simulink model "DTF"  (R2022a)
settings: Solver=FixedStepDiscrete  StartTime=0.0  StopTime=0.04  FixedStep=0.04  RelTol=1e-3
PreLoadFcn:
  | listing = dir;
  | if (contains([listing .name], 'TCAF')) && (contains([listing .name], 'MAP'))
  |     addpath('./TCAF', './MAP');
  |     addpath( genpath('./MAP') );
  | elseif (contains([listing .name], 'DTF.slx'))
  |     addpath('../TCAF', '../MAP');
  |     addpath( genpath('../MAP') );
  | else
  | end
  | 
  | load('BusStructureDTF.mat');
  | load('BusStructureWTPG.mat');
  | load('TRN\BusStructureTRN.mat');
InitFcn:
  | listing = dir;
  | if (contains([listing .name], 'TCAF')) && (contains([listing .name], 'MAP'))
  |     addpath('./TCAF', './MAP');
  |     addpath( genpath('./MAP') );
  | elseif (contains([listing .name], 'DTF.slx'))
  |     addpath('../TCAF', '../MAP');
  |     addpath( genpath('../MAP') );
  | else
  | end
  | 
  | load('BusStructureDTF.mat');
  | load('BusStructureWTPG.mat');
  | load('TRN\BusStructureTRN.mat');
StartFcn:
  | listing = dir;
  | if (contains([listing .name], 'TCAF')) && (contains([listing .name], 'MAP'))
  |     addpath('./TCAF', './MAP');
  |     addpath( genpath('./MAP') );
  | elseif (contains([listing .name], 'DTF.slx'))
  |     addpath('../TCAF', '../MAP');
  |     addpath( genpath('../MAP') );
  | else
  | end
  | 
  | load('BusStructureDTF.mat');
  | load('BusStructureWTPG.mat');
  | load('TRN\BusStructureTRN.mat');
values from neighbouring files (symbols this model uses):
  isFeasible = logsout{idx_WTPGDatapump}.Values.isFeasible.Data(ii,:)    [WTPG_SIM_AFTERPLOT.m]
undefined symbols (not defined in the file or in its folder): gLimitWarning, lowTFWarning, m, msdUsedWrap, referenceTrajectory, rideQualityWrap, s, selectedWrap, statusCode, valid, verticalGCommand
libraries: hdlsllib x15, simulink x2, aerolibconvert2 x2, simulink_extras x1
settings Model: Creator=ASCL  LastModifiedBy=ASCL
settings DataIOCC: SaveOutput=off  SignalLogging=off  DSMLogging=off  SaveTime=off  ReturnWorkspaceOutputs=off
settings OptimizationCC: BlockReduction=off  DefaultParameterBehavior=Inlined  UseDivisionForNetSlopeComputation=on  GainParamInheritBuiltInType=on  UseFloatMulNetSlope=on  ExpressionFolding=off  PassReuseOutputArgsAs=Individual arguments  ZeroExternalMemoryAtStartup=off  ZeroInternalMemoryAtStartup=off  EfficientFloat2IntCast=on  LifeSpan=inf  OptimizeBlockOrder=speed  DifferentSizesBufferReuse=on  EfficientTunableParamExpr=on
settings DebuggingCC: SignalInfNanChecking=warning  ReadBeforeWriteMsg=EnableAllAsWarning  WriteAfterWriteMsg=EnableAllAsError  WriteAfterReadMsg=EnableAllAsError  IntegerOverflowMsg=error  ParameterTunabilityLossMsg=error  UniqueDataStoreMsg=error  AssertControl=DisableAll  NonBusSignalsTreatedAsBus=error  SFInvalidInputDataAccessInChartInitDiag=error  SFTransitionOutsideNaturalParentDiag=error  SFUnreachableExecutionPathDiag=error  SFUndirectedBroadcastEventsDiag=error  IntegerSaturationMsg=error
settings HardwareCC: ProdBitPerPointer=32  ProdBitPerSizeT=32  ProdBitPerPtrDiffT=32  ProdLargestAtomicInteger=Long  ProdLargestAtomicFloat=Double  ProdEndianess=BigEndian  ProdWordSize=32  ProdLongLongMode=on  ProdHWDeviceType=Freescale->MPC83xx
settings ModelReferenceCC: ModelReferenceNumInstancesAllowed=Single
settings SFSimCC: CompileTimeRecursionLimit=0  EnableRuntimeRecursion=off  MATLABDynamicMemAlloc=off
settings RTWCC: SystemTargetFile=ert.tlc  TemplateMakefile=ert_default_tmf  GenerateReport=on  RTWUseSimCustomCode=on  BuildConfiguration=Faster Runs  IncludeHyperlinkInReport=on  LaunchReport=on  GenerateTraceInfo=on  GenerateTraceReport=on  GenerateTraceReportSl=on  GenerateTraceReportSf=on  GenerateTraceReportEml=on  GenerateCodeMetricsReport=on
settings CodeAppCC: ForceParamTrailComments=on  IgnoreCustomStorageClasses=off  OperatorAnnotations=on  SimulinkDataObjDesc=on  SFDataObjDesc=on  MATLABFcnDesc=on  InsertBlockDesc=on  StateflowObjectComments=on  MATLABSourceComments=on  EnableCustomComments=on  InlinedPrmAccess=Macros  ReqsInCode=on
settings ERTTargetCC: TargetLangStandard=C99 (ISO)  UtilityFuncGeneration=Shared location  GenerateSampleERTMain=on  IncludeMdlTerminateFcn=off  CombineSignalStateStructs=on  SuppressErrorStatus=on  SupportAbsoluteTime=off  SupportNonFinite=off  SupportComplex=off  SupportVariableSizeSignals=on  ParenthesesLevel=Standards  CastingMode=Standards  GenerateSharedConstants=off  InlinedParameterPlacement=NonHierarchical  ERTCustomFileTemplate=example_file_process.tlc  RateTransitionBlockCode=Function  PreserveIfCondition=on  ConvertIfToSwitch=off  EnableSignedLeftShifts=off  EnableSignedRightShifts=off

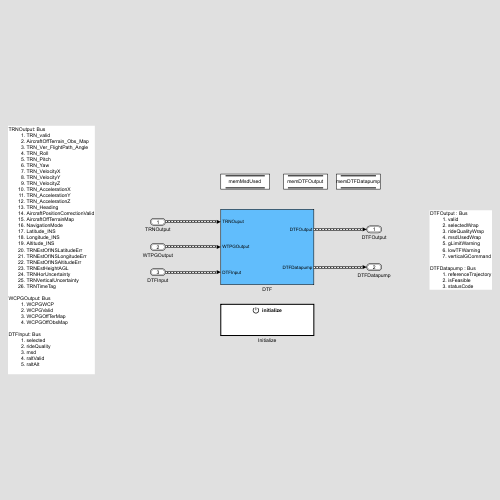
[thumbnail: Simulink's stored preview of the top-level diagram]
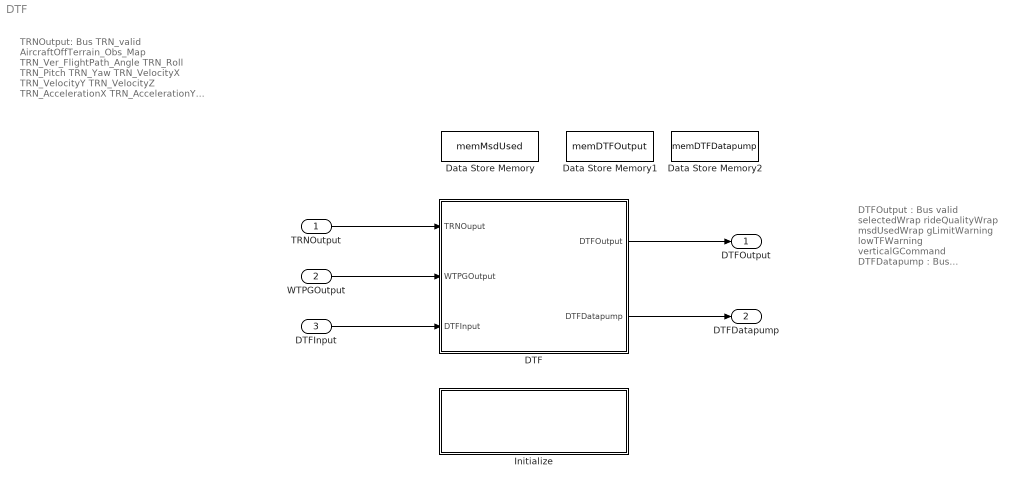
== system DTF ==
  note: TRNOutput: Bus
      | TRN_valid
      | AircraftOffTerrain_Obs_Map
      | TRN_Ver_FlightPath_Angle
      | TRN_Roll
      | TRN_Pitch
      | TRN_Yaw
      | TRN_VelocityX
      | TRN_VelocityY
      | TRN_VelocityZ
      | TRN_AccelerationX
      | TRN_AccelerationY
      | TRN_AccelerationZ
      | TRN_Heading
      | AircraftPositionCorrectionValid
      | AircraftOffTerrainMap
      | NavigationMode
      | Latitude_INS
      | Longitude_INS
      | Altitude_INS
      | TRNEstOfINSLatitudeErr
      | TRNEstOfINSLongitudeErr
      | TRNEstOfINSAltitudeErr
      | TRNEstHeightAGL
      | TRNHorUncertainty
      | TRNVerticalUncertainty
      | TRNTimeTag
      |
      | WCPGOutput: Bus
      | WCPGWCP
      | WCPGValid
      | WCPGOffTerMap
      | WCPGOffObsMap
      |
      | DTFInput: Bus
      | selected
      | rideQuality
      | msd
      | raltValid
      | raltAlt
  note: DTFOutput : Bus
      | valid
      | selectedWrap
      | rideQualityWrap
      | msdUsedWrap
      | gLimitWarning
      | lowTFWarning
      | verticalGCommand
      |
      | DTFDatapump : Bus
      | referenceTrajectory
      | isFeasible
      | statusCode
  TRNOutput : Inport  OutDataTypeStr=Bus: TRNOutput  Interpolate=off  BusOutputAsStruct=on
  WTPGOutput : Inport  Port=2  OutDataTypeStr=Bus: WTPGOutput  Interpolate=off  BusOutputAsStruct=on
  DTFInput : Inport  Port=3  OutDataTypeStr=Bus: DTFInput  Interpolate=off  BusOutputAsStruct=on
  DTF : Subsystem
  Data Store Memory : DataStoreMemory  DataStoreName=memMsdUsed  WriteAfterWriteMsg=warning  ShowAdditionalParam=off  OutDataTypeStr=double
      settings: LockScale=on
  Data Store Memory1 : DataStoreMemory  DataStoreName=memDTFOutput  WriteAfterWriteMsg=warning  ShowAdditionalParam=off  OutDataTypeStr=Bus: DTFOutput
      settings: LockScale=on
  Data Store Memory2 : DataStoreMemory  DataStoreName=memDTFDatapump  WriteAfterWriteMsg=warning  ShowAdditionalParam=off  OutDataTypeStr=Bus: DTFDatapump
      settings: LockScale=on
  Initialize : Subsystem  TreatAsAtomicUnit=on
  DTFOutput : Outport  OutDataTypeStr=Bus: DTFOutput  SampleTime=0.04  BusOutputAsStruct=on
  DTFDatapump : Outport  Port=2  OutDataTypeStr=Bus: DTFDatapump  SampleTime=0.04  BusOutputAsStruct=on
  wires:
  TRNOutput/1 -> DTF/1(TRNOuput)
  WTPGOutput/1 -> DTF/2(WTPGOutput)
  DTFInput/1 -> DTF/3(DTFInput)
  DTF/1(DTFOutput) -> DTFOutput/1
  DTF/2(DTFDatapump) -> DTFDatapump/1

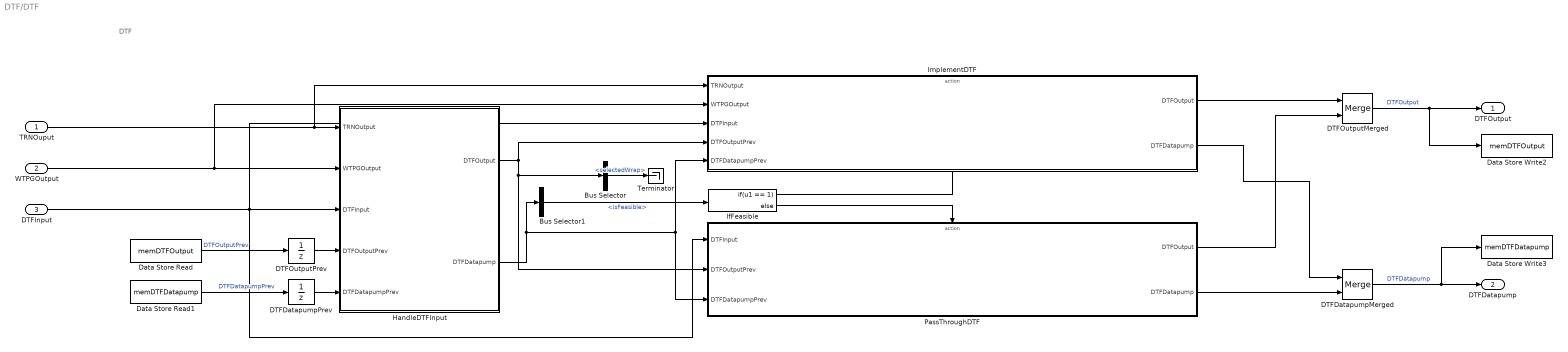
== system DTF/DTF ==
  note: DTF
  TRNOuput : Inport  OutDataTypeStr=Bus: TRNOutput
  WTPGOutput : Inport  Port=2  OutDataTypeStr=Bus: WTPGOutput
  DTFInput : Inport  Port=3  OutDataTypeStr=Bus: DTFInput
  Bus Selector : BusSelector  OutputSignals=selectedWrap
  Bus Selector1 : BusSelector  OutputSignals=isFeasible
  DTFDatapumpMerged : Merge
  DTFDatapumpPrev : UnitDelay  SampleTime=-1  HasFrameUpgradeWarning=on
  DTFOutputMerged : Merge
  DTFOutputPrev : UnitDelay  SampleTime=-1  HasFrameUpgradeWarning=on
  Data Store Read : DataStoreRead  DataStoreName=memDTFOutput  IndexOptions=Index vector (dialog)  Indices=1  OutputSizes=1
  Data Store Read1 : DataStoreRead  DataStoreName=memDTFDatapump  IndexOptions=Index vector (dialog)  Indices=1  OutputSizes=1
  Data Store Write2 : DataStoreWrite  DataStoreName=memDTFOutput  IndexOptions=Index vector (dialog)  Indices=1  OutputSizes=1
  Data Store Write3 : DataStoreWrite  DataStoreName=memDTFDatapump  IndexOptions=Index vector (dialog)  Indices=1  OutputSizes=1
  HandleDTFInput : Subsystem  TreatAsAtomicUnit=on
      settings: RTWSystemCode=Nonreusable function  RTWFcnNameOpts=Use subsystem name
  IfFeasible : If  IfExpression=u1 == 1
  ImplementDTF : Subsystem  TreatAsAtomicUnit=on
      settings: RTWSystemCode=Nonreusable function  RTWFcnNameOpts=Use subsystem name
  PassThroughDTF : Subsystem  TreatAsAtomicUnit=on
      settings: RTWSystemCode=Nonreusable function  RTWFcnNameOpts=Use subsystem name
  Terminator : Terminator
  DTFOutput : Outport  OutDataTypeStr=Bus: DTFOutput
  DTFDatapump : Outport  Port=2  OutDataTypeStr=Bus: DTFDatapump
  wires:
  ImplementDTF/1(DTFOutput) -> DTFOutputMerged/1
  PassThroughDTF/1(DTFOutput) -> DTFOutputMerged/2
  DTFOutputPrev/1 -> HandleDTFInput/4(DTFOutputPrev)
  IfFeasible/2 -> PassThroughDTF/Action
  TRNOuput/1 -> ImplementDTF/1(TRNOutput), HandleDTFInput/1(TRNOutput)
  Data Store Read/1 -> DTFOutputPrev/1  "DTFOutputPrev"
  DTFDatapumpPrev/1 -> HandleDTFInput/5(DTFDatapumpPrev)
  WTPGOutput/1 -> ImplementDTF/2(WTPGOutput), HandleDTFInput/2(WTPGOutput)
  ImplementDTF/2(DTFDatapump) -> DTFDatapumpMerged/1
  DTFInput/1 -> PassThroughDTF/1(DTFInput), ImplementDTF/3(DTFInput), HandleDTFInput/3(DTFInput)
  HandleDTFInput/2(DTFDatapump) -> Bus Selector1/1, PassThroughDTF/3(DTFDatapumpPrev), ImplementDTF/5(DTFDatapumpPrev)
  PassThroughDTF/2(DTFDatapump) -> DTFDatapumpMerged/2
  IfFeasible/1 -> ImplementDTF/Action
  Data Store Read1/1 -> DTFDatapumpPrev/1  "DTFDatapumpPrev"
  Bus Selector1/1 -> IfFeasible/1  "<isFeasible>"
  DTFOutputMerged/1 -> Data Store Write2/1, DTFOutput/1  "DTFOutput"
  DTFDatapumpMerged/1 -> Data Store Write3/1, DTFDatapump/1  "DTFDatapump"
  HandleDTFInput/1(DTFOutput) -> PassThroughDTF/2(DTFOutputPrev), Bus Selector/1, ImplementDTF/4(DTFOutputPrev)
  Bus Selector/1 -> Terminator/1  "<selectedWrap>"

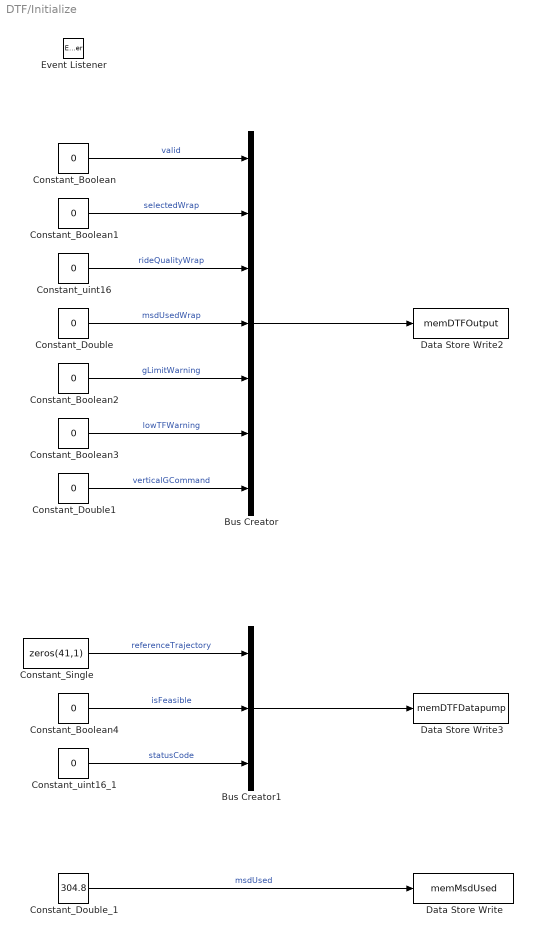
== system DTF/Initialize ==
  Bus Creator : BusCreator  Inputs=7  OutDataTypeStr=Bus: DTFOutput  NonVirtualBus=on
  Bus Creator1 : BusCreator  Inputs=3  OutDataTypeStr=Bus: DTFDatapump  NonVirtualBus=on
  Constant_Boolean{,1..4} (5 alike) : Constant  Value=0  OutDataTypeStr=boolean
  Constant_Double : Constant  Value=0  OutDataTypeStr=double
  Constant_Double1 : Constant  Value=0  OutDataTypeStr=double
  Constant_Double_1 : Constant  Value=304.8  VectorParams1D=off  OutDataTypeStr=double
  Constant_Single : Constant  Value=zeros(41,1)  OutDataTypeStr=single
  Constant_uint16 : Constant  Value=0  OutDataTypeStr=uint16
  Constant_uint16_1 : Constant  Value=0  OutDataTypeStr=uint16
  Data Store Write : DataStoreWrite  DataStoreName=memMsdUsed  IndexOptions=Index vector (dialog)  Indices=1  OutputSizes=1
  Data Store Write2 : DataStoreWrite  DataStoreName=memDTFOutput  IndexOptions=Index vector (dialog)  Indices=1  OutputSizes=1
  Data Store Write3 : DataStoreWrite  DataStoreName=memDTFDatapump  IndexOptions=Index vector (dialog)  Indices=1  OutputSizes=1
  Event Listener : EventListener  DisableCoverage=on  EventName=reset
  wires:
  Constant_Boolean/1 -> Bus Creator/1  "valid"
  Constant_Boolean1/1 -> Bus Creator/2  "selectedWrap"
  Constant_Boolean3/1 -> Bus Creator/6  "lowTFWarning"
  Constant_Boolean2/1 -> Bus Creator/5  "gLimitWarning"
  Constant_Double/1 -> Bus Creator/4  "msdUsedWrap"
  Constant_Double1/1 -> Bus Creator/7  "verticalGCommand"
  Constant_uint16/1 -> Bus Creator/3  "rideQualityWrap"
  Bus Creator/1 -> Data Store Write2/1
  Bus Creator1/1 -> Data Store Write3/1
  Constant_uint16_1/1 -> Bus Creator1/3  "statusCode"
  Constant_Boolean4/1 -> Bus Creator1/2  "isFeasible"
  Constant_Single/1 -> Bus Creator1/1  "referenceTrajectory"
  Constant_Double_1/1 -> Data Store Write/1  "msdUsed"

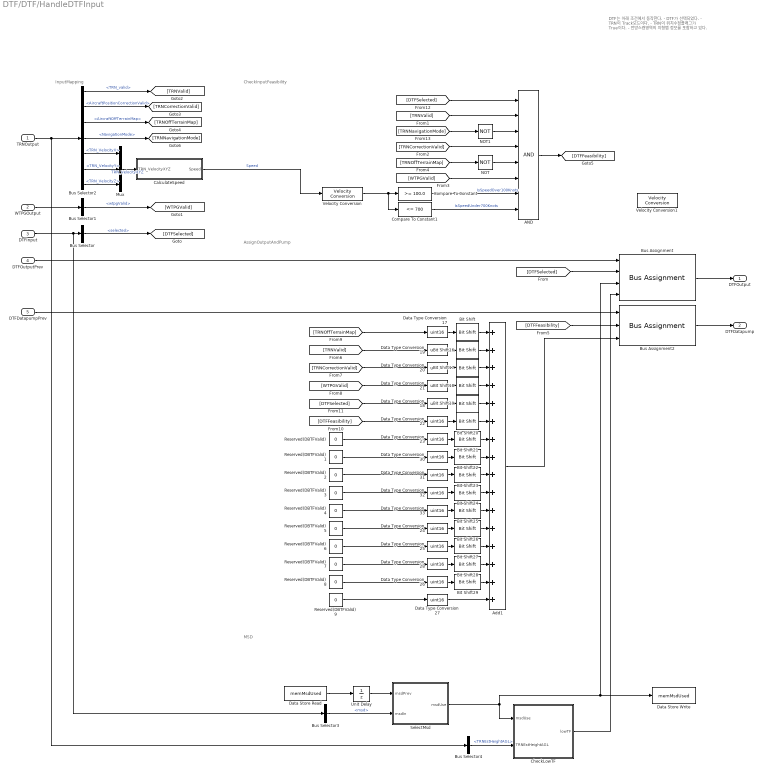
== system DTF/DTF/HandleDTFInput ==
  note: MSD
  note: AssignOutputAndPump
  note: DTF는 아래 조건에서 동작한다.
      | - DTF가 선택되었다.
      | - TRN이 Track모드이다.
      | - TRN이 위치수정플래그가 True이다.
      | - 전방스캔영역의 지형맵 정보를 포함하고 있다.
  note: CheckInputFeasibility
  note: InputMapping
  TRNOutput : Inport  OutDataTypeStr=Bus: TRNOutput
  WTPGOutput : Inport  Port=2  OutDataTypeStr=Bus: WTPGOutput
  DTFInput : Inport  Port=3  OutDataTypeStr=Bus: DTFInput
  DTFOutputPrev : Inport  Port=4  OutDataTypeStr=Bus: DTFOutput
  DTFDatapumpPrev : Inport  Port=5  OutDataTypeStr=Bus: DTFDatapump
  AND : Logic  Inputs=8  AllPortsSameDT=off  OutDataTypeStr=boolean
  Add1 : Sum  Inputs=++++++++++++++++  AccumDataTypeStr=uint16
  Bit Shift : hdlsllib/Logic and Bit Operations/Bit Shift  mode=Shift Left Logical  N=15
  Bit Shift16 : hdlsllib/Logic and Bit Operations/Bit Shift  mode=Shift Left Logical  N=14
  Bit Shift17 : hdlsllib/Logic and Bit Operations/Bit Shift  mode=Shift Left Logical  N=13
  Bit Shift18 : hdlsllib/Logic and Bit Operations/Bit Shift  mode=Shift Left Logical  N=12
  Bit Shift19 : hdlsllib/Logic and Bit Operations/Bit Shift  mode=Shift Left Logical  N=11
  Bit Shift20 : hdlsllib/Logic and Bit Operations/Bit Shift  mode=Shift Left Logical  N=10
  Bit Shift21 : hdlsllib/Logic and Bit Operations/Bit Shift  mode=Shift Left Logical  N=9
  Bit Shift22 : hdlsllib/Logic and Bit Operations/Bit Shift  mode=Shift Left Logical  N=8
  Bit Shift23 : hdlsllib/Logic and Bit Operations/Bit Shift  mode=Shift Left Logical  N=7
  Bit Shift24 : hdlsllib/Logic and Bit Operations/Bit Shift  mode=Shift Left Logical  N=6
  Bit Shift25 : hdlsllib/Logic and Bit Operations/Bit Shift  mode=Shift Left Logical  N=5
  Bit Shift26 : hdlsllib/Logic and Bit Operations/Bit Shift  mode=Shift Left Logical  N=4
  Bit Shift27 : hdlsllib/Logic and Bit Operations/Bit Shift  mode=Shift Left Logical  N=3
  Bit Shift28 : hdlsllib/Logic and Bit Operations/Bit Shift  mode=Shift Left Logical  N=2
  Bit Shift29 : hdlsllib/Logic and Bit Operations/Bit Shift  mode=Shift Left Logical  N=1
  Bus Assignment : BusAssignment  AssignedSignals=selectedWrap,msdUsedWrap,lowTFWarning
  Bus Assignment2 : BusAssignment  AssignedSignals=isFeasible,statusCode
  Bus Selector : BusSelector  OutputSignals=selected
  Bus Selector1 : BusSelector  OutputSignals=wtpgValid
  Bus Selector2 : BusSelector  OutputSignals=TRN_valid,AircraftPositionCorrectionValid,AircraftOffTerrainMap,NavigationMode,TRN_VelocityX,TRN_VelocityY,TRN_VelocityZ
  Bus Selector3 : BusSelector  OutputSignals=msd
  Bus Selector4 : BusSelector  OutputSignals=TRNEstHeightAGL
  CalculateSpeed : Subsystem
  CheckLowTF : MATLAB Function  TreatAsAtomicUnit=on
      settings: RTWSystemCode=Nonreusable function  RTWFcnNameOpts=Use subsystem name  FunctionInterfaceSpec=Allow arguments (Match graphical interface)
  Compare To Constant : simulink/Logic and Bit Operations/Compare To Constant  relop=>=  const=100.0  OutDataTypeStr=boolean
  Compare To Constant1 : simulink/Logic and Bit Operations/Compare To Constant  relop=<=  const=700  OutDataTypeStr=boolean
  Data Store Read : DataStoreRead  DataStoreName=memMsdUsed  IndexOptions=Index vector (dialog)  Indices=1  OutputSizes=1
  Data Store Write : DataStoreWrite  DataStoreName=memMsdUsed  IndexOptions=Index vector (dialog)  Indices=1  OutputSizes=1
  Data Type Conversion{17..28,30..33} (16 alike) : DataTypeConversion  OutDataTypeStr=uint16  SaturateOnIntegerOverflow=off  RndMeth=Floor
  Mux : Mux  Inputs=3
  NOT : Logic  Operator=NOT  AllPortsSameDT=off  OutDataTypeStr=boolean
  NOT1 : Logic  Operator=NOT  AllPortsSameDT=off  OutDataTypeStr=boolean
  Reserved(DBTFValid){,1..9} (10 alike) : Constant  Value=0  OutDataTypeStr=boolean
  SelectMsd : MATLAB Function  TreatAsAtomicUnit=on
      settings: RTWSystemCode=Nonreusable function  RTWFcnNameOpts=Use subsystem name  FunctionInterfaceSpec=Allow arguments (Match graphical interface)
  Unit Delay : UnitDelay  SampleTime=-1  HasFrameUpgradeWarning=on
  Velocity Conversion : aerolibconvert2/Velocity Conversion  IU=m/s  OU=kts
  Velocity Conversion1 : aerolibconvert2/Velocity Conversion  IU=m/s  OU=kts
  DTFOutput : Outport  OutDataTypeStr=Bus: DTFOutput  VectorParamsAs1DForOutWhenUnconnected=off
  DTFDatapump : Outport  Port=2  OutDataTypeStr=Bus: DTFDatapump  VectorParamsAs1DForOutWhenUnconnected=off
  wires:
  DTFInput/1 -> Bus Selector3/1, Bus Selector/1
  DTFOutputPrev/1 -> Bus Assignment/1
  Bus Assignment/1 -> DTFOutput/1
  DTFDatapumpPrev/1 -> Bus Assignment2/1
  WTPGOutput/1 -> Bus Selector1/1
  TRNOutput/1 -> Bus Selector4/1, Bus Selector2/1
  Bus Selector2/2 -> [TRNCorrectionValid]  "<AircraftPositionCorrectionValid>"
  Bus Selector2/3 -> [TRNOffTerrainMap]  "<AircraftOffTerrainMap>"
  Bus Selector/1 -> [DTFSelected]  "<selected>"
  Bus Selector1/1 -> [WTPGValid]  "<wtpgValid>"
  Bus Selector2/1 -> [TRNValid]  "<TRN_valid>"
  [DTFSelected] -> Bus Assignment/2
  [TRNOffTerrainMap] -> NOT/1
  Bus Assignment2/1 -> DTFDatapump/1
  Add1/1 -> Bus Assignment2/3
  [TRNOffTerrainMap] -> Data Type Conversion17/1
  [TRNCorrectionValid] -> Data Type Conversion20/1
  [WTPGValid] -> Data Type Conversion21/1
  [DTFFeasibility] -> Data Type Conversion22/1
  [DTFSelected] -> Data Type Conversion18/1
  Reserved(DBTFValid)/1 -> Data Type Conversion23/1
  [TRNValid] -> Data Type Conversion19/1
  AND/1 -> [DTFFeasibility]
  [DTFSelected] -> AND/1
  Bus Selector2/4 -> [TRNNavigationMode]  "<NavigationMode>"
  [TRNValid] -> AND/2
  [TRNNavigationMode] -> NOT1/1
  [TRNCorrectionValid] -> AND/4
  [WTPGValid] -> AND/6
  NOT/1 -> AND/5
  Data Type Conversion18/1 -> Bit Shift19/1
  Bit Shift/1 -> Add1/1
  Data Type Conversion27/1 -> Add1/16
  Data Type Conversion26/1 -> Bit Shift29/1
  Bit Shift29/1 -> Add1/15
  Data Type Conversion33/1 -> Bit Shift25/1
  Data Type Conversion22/1 -> Bit Shift20/1
  Data Type Conversion20/1 -> Bit Shift17/1
  Data Type Conversion24/1 -> Bit Shift26/1
  Data Type Conversion19/1 -> Bit Shift16/1
  Bit Shift28/1 -> Add1/14
  Data Type Conversion32/1 -> Bit Shift24/1
  Data Type Conversion23/1 -> Bit Shift21/1
  Bit Shift23/1 -> Add1/9
  Data Type Conversion25/1 -> Bit Shift27/1
  Data Type Conversion30/1 -> Bit Shift22/1
  Data Type Conversion17/1 -> Bit Shift/1
  Data Type Conversion31/1 -> Bit Shift23/1
  Bit Shift24/1 -> Add1/10
  Data Type Conversion28/1 -> Bit Shift28/1
  Bit Shift25/1 -> Add1/11
  Data Type Conversion21/1 -> Bit Shift18/1
  Bit Shift27/1 -> Add1/13
  Bit Shift21/1 -> Add1/7
  Bit Shift19/1 -> Add1/5
  Bit Shift20/1 -> Add1/6
  Bit Shift22/1 -> Add1/8
  Bit Shift18/1 -> Add1/4
  Bit Shift17/1 -> Add1/3
  Bit Shift16/1 -> Add1/2
  Bit Shift26/1 -> Add1/12
  [DTFFeasibility] -> Bus Assignment2/2
  Reserved(DBTFValid)9/1 -> Data Type Conversion27/1
  Reserved(DBTFValid)8/1 -> Data Type Conversion26/1
  Reserved(DBTFValid)7/1 -> Data Type Conversion28/1
  Reserved(DBTFValid)6/1 -> Data Type Conversion25/1
  Reserved(DBTFValid)1/1 -> Data Type Conversion30/1
  Reserved(DBTFValid)2/1 -> Data Type Conversion31/1
  Reserved(DBTFValid)3/1 -> Data Type Conversion32/1
  Reserved(DBTFValid)4/1 -> Data Type Conversion33/1
  Reserved(DBTFValid)5/1 -> Data Type Conversion24/1
  NOT1/1 -> AND/3
  Bus Selector3/1 -> SelectMsd/2(msdIn)  "<msd>"
  Data Store Read/1 -> Unit Delay/1
  Unit Delay/1 -> SelectMsd/1(msdPrev)
  SelectMsd/1(msdUse) -> Data Store Write/1, Bus Assignment/3, CheckLowTF/1(msdUse)
  CheckLowTF/1(lowTF) -> Bus Assignment/4
  Bus Selector2/5 -> Mux/1  "<TRN_VelocityX>"
  Bus Selector2/6 -> Mux/2  "<TRN_VelocityY>"
  Bus Selector2/7 -> Mux/3  "<TRN_VelocityZ>"
  Mux/1 -> CalculateSpeed/1(TRN_VelocityXYZ)  "TRN_VelocityXYZ"
  Compare To Constant/1 -> AND/7  "IsSpeedOver100Knots"
  CalculateSpeed/1(Speed) -> Velocity Conversion/1  "Speed"
  Compare To Constant1/1 -> AND/8  "IsSpeedUnder700Knots"
  Bus Selector4/1 -> CheckLowTF/2(TRNEstHeightAGL)  "<TRNEstHeightAGL>"
  Velocity Conversion/1 -> Compare To Constant1/1, Compare To Constant/1

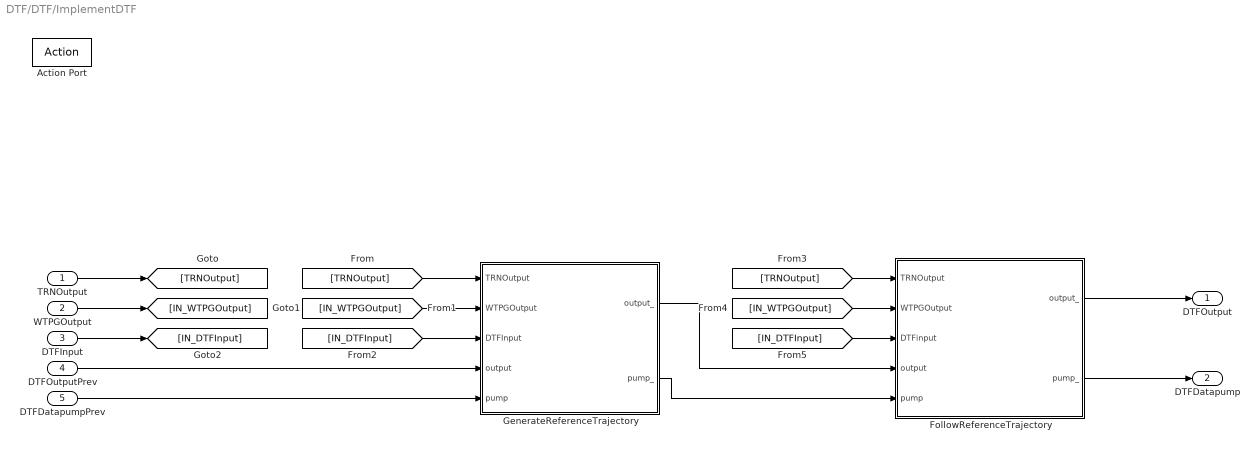
== system DTF/DTF/ImplementDTF ==
  TRNOutput : Inport  OutDataTypeStr=Bus: TRNOutput
  WTPGOutput : Inport  Port=2  OutDataTypeStr=Bus: WTPGOutput
  DTFInput : Inport  Port=3  OutDataTypeStr=Bus: DTFInput
  DTFOutputPrev : Inport  Port=4  OutDataTypeStr=Bus: DTFOutput
  DTFDatapumpPrev : Inport  Port=5  OutDataTypeStr=Bus: DTFDatapump
  Action Port : ActionPort  ActionPortLabel=if(u1 == 1)
  FollowReferenceTrajectory : Subsystem  TreatAsAtomicUnit=on
      settings: RTWSystemCode=Nonreusable function  RTWFcnNameOpts=Use subsystem name
  GenerateReferenceTrajectory : Subsystem  TreatAsAtomicUnit=on
      settings: RTWSystemCode=Nonreusable function  RTWFcnNameOpts=Use subsystem name
  DTFOutput : Outport  OutDataTypeStr=Bus: DTFOutput  VectorParamsAs1DForOutWhenUnconnected=off
  DTFDatapump : Outport  Port=2  OutDataTypeStr=Bus: DTFDatapump  VectorParamsAs1DForOutWhenUnconnected=off
  wires:
  DTFInput/1 -> [IN_DTFInput]
  FollowReferenceTrajectory/2(pump_) -> DTFDatapump/1
  FollowReferenceTrajectory/1(output_) -> DTFOutput/1
  TRNOutput/1 -> [TRNOutput]
  WTPGOutput/1 -> [IN_WTPGOutput]
  [TRNOutput] -> FollowReferenceTrajectory/1(TRNOutput)
  [IN_WTPGOutput] -> FollowReferenceTrajectory/2(WTPGOutput)
  [IN_DTFInput] -> FollowReferenceTrajectory/3(DTFinput)
  [TRNOutput] -> GenerateReferenceTrajectory/1(TRNOutput)
  [IN_WTPGOutput] -> GenerateReferenceTrajectory/2(WTPGOutput)
  [IN_DTFInput] -> GenerateReferenceTrajectory/3(DTFInput)
  DTFOutputPrev/1 -> GenerateReferenceTrajectory/4(output)
  DTFDatapumpPrev/1 -> GenerateReferenceTrajectory/5(pump)
  GenerateReferenceTrajectory/1(output_) -> FollowReferenceTrajectory/4(output)
  GenerateReferenceTrajectory/2(pump_) -> FollowReferenceTrajectory/5(pump)

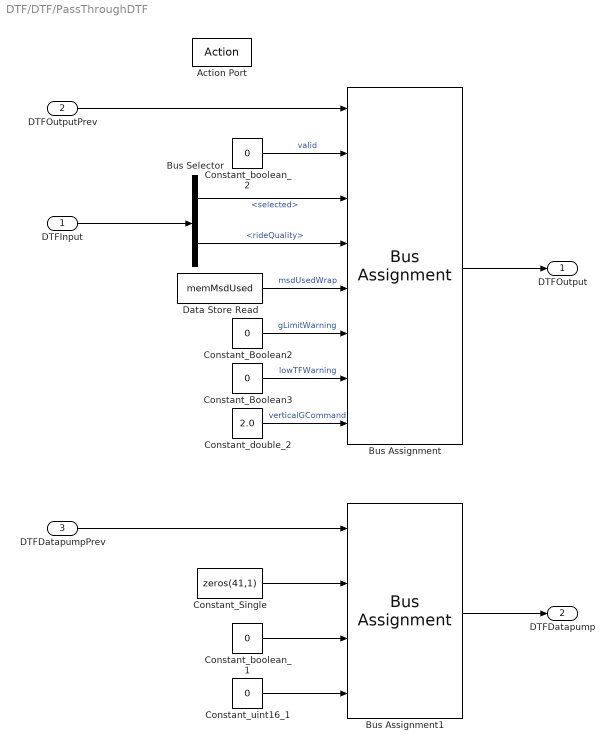
== system DTF/DTF/PassThroughDTF ==
  DTFInput : Inport  OutDataTypeStr=Bus: DTFInput
  DTFOutputPrev : Inport  Port=2  OutDataTypeStr=Bus: DTFOutput
  DTFDatapumpPrev : Inport  Port=3  OutDataTypeStr=Bus: DTFDatapump
  Action Port : ActionPort  ActionPortLabel=else
  Bus Assignment : BusAssignment  AssignedSignals=valid,selectedWrap,rideQualityWrap,msdUsedWrap,gLimitWarning,lowTFWarning,verticalGCommand
  Bus Assignment1 : BusAssignment  AssignedSignals=referenceTrajectory,isFeasible,statusCode
  Bus Selector : BusSelector  OutputSignals=selected,rideQuality
  Constant_Boolean2 : Constant  Value=0  OutDataTypeStr=boolean
  Constant_Boolean3 : Constant  Value=0  OutDataTypeStr=boolean
  Constant_Single : Constant  Value=zeros(41,1)  OutDataTypeStr=single
  Constant_boolean_1 : Constant  Value=0  OutDataTypeStr=boolean
  Constant_boolean_2 : Constant  Value=0  OutDataTypeStr=boolean
  Constant_double_2 : Constant  Value=2.0  OutDataTypeStr=double
  Constant_uint16_1 : Constant  Value=0  OutDataTypeStr=uint16
  Data Store Read : DataStoreRead  DataStoreName=memMsdUsed  IndexOptions=Index vector (dialog)  Indices=1  OutputSizes=1
  DTFOutput : Outport  OutDataTypeStr=Bus: DTFOutput  VectorParamsAs1DForOutWhenUnconnected=off
  DTFDatapump : Outport  Port=2  OutDataTypeStr=Bus: DTFDatapump  VectorParamsAs1DForOutWhenUnconnected=off
  wires:
  DTFOutputPrev/1 -> Bus Assignment/1
  DTFDatapumpPrev/1 -> Bus Assignment1/1
  Bus Assignment/1 -> DTFOutput/1
  Bus Assignment1/1 -> DTFDatapump/1
  Constant_Single/1 -> Bus Assignment1/2
  Constant_boolean_1/1 -> Bus Assignment1/3
  Constant_uint16_1/1 -> Bus Assignment1/4
  Constant_boolean_2/1 -> Bus Assignment/2  "valid"
  Constant_Boolean3/1 -> Bus Assignment/7  "lowTFWarning"
  Constant_double_2/1 -> Bus Assignment/8  "verticalGCommand"
  Data Store Read/1 -> Bus Assignment/5  "msdUsedWrap"
  Constant_Boolean2/1 -> Bus Assignment/6  "gLimitWarning"
  Bus Selector/1 -> Bus Assignment/3  "<selected>"
  Bus Selector/2 -> Bus Assignment/4  "<rideQuality>"
  DTFInput/1 -> Bus Selector/1

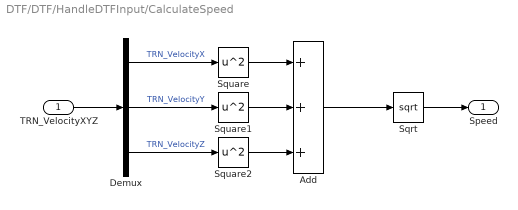
== system DTF/DTF/HandleDTFInput/CalculateSpeed ==
  TRN_VelocityXYZ : Inport
  Add : Sum  Inputs=+++
  Demux : Demux  Outputs=3
  Sqrt : Sqrt
  Square : Math  Operator=square  SignedPower=on  RndMeth=Zero
  Square1 : Math  Operator=square  SignedPower=on  RndMeth=Zero
  Square2 : Math  Operator=square  SignedPower=on  RndMeth=Zero
  Speed : Outport
  wires:
  Demux/1 -> Square/1  "TRN_VelocityX"
  Demux/3 -> Square2/1  "TRN_VelocityZ"
  Demux/2 -> Square1/1  "TRN_VelocityY"
  Square/1 -> Add/1
  Square1/1 -> Add/2
  Square2/1 -> Add/3
  Add/1 -> Sqrt/1
  Sqrt/1 -> Speed/1
  TRN_VelocityXYZ/1 -> Demux/1

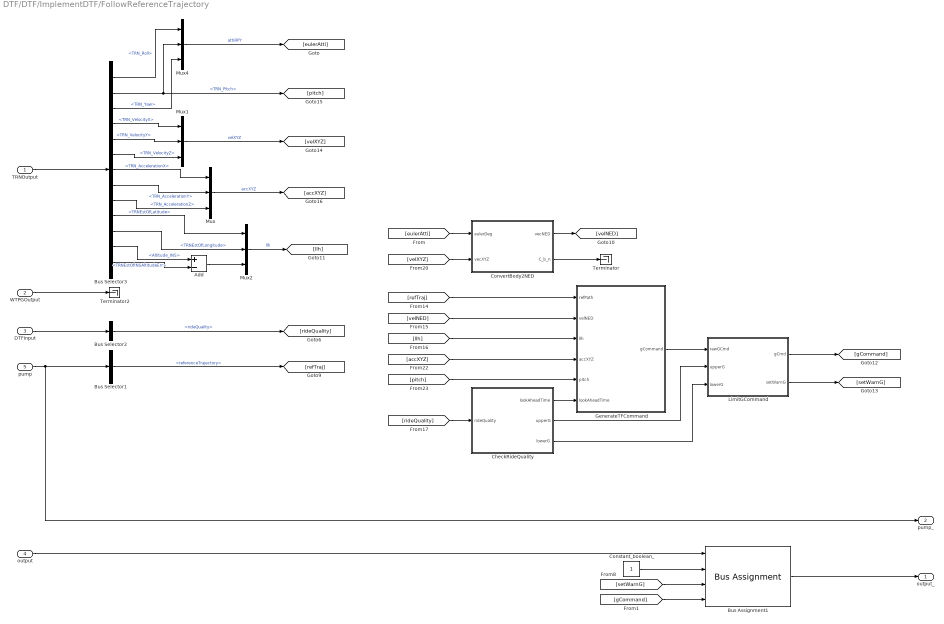
== system DTF/DTF/ImplementDTF/FollowReferenceTrajectory ==
  TRNOutput : Inport  OutDataTypeStr=Bus: TRNOutput
  WTPGOutput : Inport  Port=2  OutDataTypeStr=Bus: WTPGOutput
  DTFinput : Inport  Port=3  OutDataTypeStr=Bus: DTFInput
  output : Inport  Port=4  OutDataTypeStr=Bus: DTFOutput
  pump : Inport  Port=5  OutDataTypeStr=Bus: DTFDatapump
  Add : Sum  Inputs=+-
  Bus Assignment1 : BusAssignment  AssignedSignals=valid,gLimitWarning,verticalGCommand
  Bus Selector1 : BusSelector  OutputSignals=referenceTrajectory
  Bus Selector2 : BusSelector  OutputSignals=rideQuality
  Bus Selector3 : BusSelector  OutputSignals=TRN_Roll,TRN_Pitch,TRN_Yaw,TRN_VelocityX,TRN_VelocityY,TRN_VelocityZ,TRN_AccelerationX,TRN_AccelerationY,TRN_AccelerationZ,TRNEstOfLatitude,TRNEstOfLongitude,Altitude_INS,TRNEstOfINSAltitudeErr
  CheckRideQuality : MATLAB Function  TreatAsAtomicUnit=on
      settings: RTWSystemCode=Nonreusable function  RTWFcnNameOpts=Use subsystem name  FunctionInterfaceSpec=Allow arguments (Match graphical interface)
  Constant_boolean_ : Constant  OutDataTypeStr=boolean
  ConvertBody2NED : MATLAB Function  TreatAsAtomicUnit=on
  GenerateTFCommand : MATLAB Function  TreatAsAtomicUnit=on
      settings: RTWSystemCode=Nonreusable function  RTWFcnNameOpts=Use subsystem name  FunctionInterfaceSpec=Allow arguments (Match graphical interface)
  LimitGCommand : MATLAB Function  TreatAsAtomicUnit=on
      settings: RTWSystemCode=Nonreusable function  RTWFcnNameOpts=Use subsystem name  FunctionInterfaceSpec=Allow arguments (Match graphical interface)
  Mux{,1..2,4} (4 alike) : Mux  Inputs=3
  Terminator : Terminator
  Terminator2 : Terminator
  output_ : Outport  OutDataTypeStr=Bus: DTFOutput  VectorParamsAs1DForOutWhenUnconnected=off
  pump_ : Outport  Port=2  OutDataTypeStr=Bus: DTFDatapump  VectorParamsAs1DForOutWhenUnconnected=off
  wires:
  DTFinput/1 -> Bus Selector2/1
  pump/1 -> pump_/1, Bus Selector1/1
  output/1 -> Bus Assignment1/1
  Bus Selector2/1 -> [rideQuality]  "<rideQuality>"
  [llh] -> GenerateTFCommand/3(llh)
  [velNED] -> GenerateTFCommand/2(velNED)
  [refTraj] -> GenerateTFCommand/1(refPath)
  [rideQuality] -> CheckRideQuality/1(rideQuality)
  [pitch] -> GenerateTFCommand/5(pitch)
  [accXYZ] -> GenerateTFCommand/4(accXYZ)
  [setWarnG] -> Bus Assignment1/3
  [gCommand] -> Bus Assignment1/4
  Bus Assignment1/1 -> output_/1
  WTPGOutput/1 -> Terminator2/1
  TRNOutput/1 -> Bus Selector3/1
  Bus Selector3/7 -> Mux/1  "<TRN_AccelerationX>"
  Bus Selector3/8 -> Mux/2  "<TRN_AccelerationY>"
  Bus Selector3/9 -> Mux/3  "<TRN_AccelerationZ>"
  Bus Selector3/4 -> Mux1/1  "<TRN_VelocityX>"
  Bus Selector3/5 -> Mux1/2  "<TRN_VelocityY>"
  Bus Selector3/6 -> Mux1/3  "<TRN_VelocityZ>"
  Mux/1 -> [accXYZ]  "accXYZ"
  Mux1/1 -> [velXYZ]  "velXYZ"
  Bus Selector1/1 -> [refTraj]  "<referenceTrajectory>"
  Mux2/1 -> [llh]  "llh"
  Bus Selector3/3 -> Mux4/3  "<TRN_Yaw>"
  Bus Selector3/1 -> Mux4/1  "<TRN_Roll>"
  Bus Selector3/2 -> Mux4/2, [pitch]  "<TRN_Pitch>"
  Mux4/1 -> [eulerAtti]  "attiRPY"
  ConvertBody2NED/1(vecNED) -> [velNED]
  [eulerAtti] -> ConvertBody2NED/1(eulerDeg)
  [velXYZ] -> ConvertBody2NED/2(vecXYZ)
  ConvertBody2NED/2(C_b_n) -> Terminator/1
  Bus Selector3/10 -> Mux2/1  "<TRNEstOfLatitude>"
  Bus Selector3/11 -> Mux2/2  "<TRNEstOfLongitude>"
  Bus Selector3/12 -> Add/1  "<Altitude_INS>"
  Bus Selector3/13 -> Add/2  "<TRNEstOfINSAltitudeErr>"
  Add/1 -> Mux2/3
  CheckRideQuality/1(lookAheadTime) -> GenerateTFCommand/6(lookAheadTime)
  CheckRideQuality/2(upperG) -> LimitGCommand/2(upperG)
  CheckRideQuality/3(lowerG) -> LimitGCommand/3(lowerG)
  GenerateTFCommand/1(gCommand) -> LimitGCommand/1(rawGCmd)
  LimitGCommand/1(gCmd) -> [gCommand]
  LimitGCommand/2(setWarnG) -> [setWarnG]
  Constant_boolean_/1 -> Bus Assignment1/2

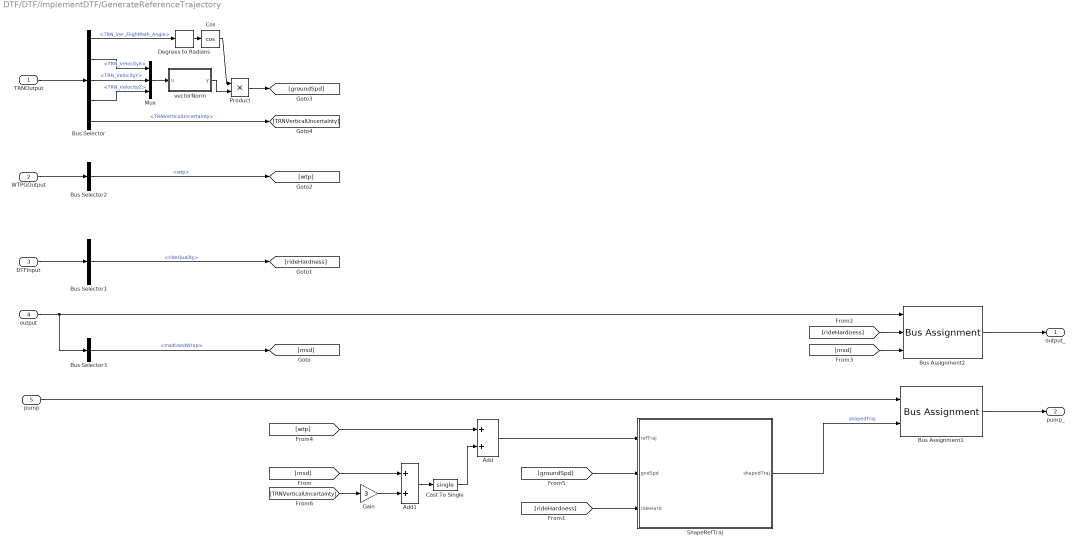
== system DTF/DTF/ImplementDTF/GenerateReferenceTrajectory ==
  TRNOutput : Inport  OutDataTypeStr=Bus: TRNOutput
  WTPGOutput : Inport  Port=2  OutDataTypeStr=Bus: WTPGOutput
  DTFInput : Inport  Port=3  OutDataTypeStr=Bus: DTFInput
  output : Inport  Port=4  OutDataTypeStr=Bus: DTFOutput
  pump : Inport  Port=5  OutDataTypeStr=Bus: DTFDatapump
  Add : Sum
  Add1 : Sum
  Bus Assignment1 : BusAssignment  AssignedSignals=referenceTrajectory
  Bus Assignment2 : BusAssignment  AssignedSignals=rideQualityWrap,msdUsedWrap
  Bus Selector : BusSelector  OutputSignals=TRN_Ver_FlightPath_Angle,TRN_VelocityX,TRN_VelocityY,TRN_VelocityZ,TRNVerticalUncertainty
  Bus Selector1 : BusSelector  OutputSignals=rideQuality
  Bus Selector2 : BusSelector  OutputSignals=wtp
  Bus Selector3 : BusSelector  OutputSignals=msdUsedWrap
  Cast To Single : DataTypeConversion  OutDataTypeStr=single  SaturateOnIntegerOverflow=off  RndMeth=Floor
  Cos : Trigonometry  Operator=cos
  Degrees to Radians : simulink_extras/Transformations/Degrees to Radians
  Gain : Gain  Gain=3
  Mux : Mux  Inputs=3
  Product : Product
  ShapeRefTraj : MATLAB Function  TreatAsAtomicUnit=on
  vectorNorm : MATLAB Function  TreatAsAtomicUnit=on
  output_ : Outport  OutDataTypeStr=Bus: DTFOutput  VectorParamsAs1DForOutWhenUnconnected=off
  pump_ : Outport  Port=2  OutDataTypeStr=Bus: DTFDatapump  VectorParamsAs1DForOutWhenUnconnected=off
  wires:
  Product/1 -> [groundSpd]
  Bus Selector/5 -> [TRNVerticalUncertainty]  "<TRNVerticalUncertainty>"
  ShapeRefTraj/1(shapedTraj) -> Bus Assignment1/2  "shapedTraj"
  [rideHardness] -> ShapeRefTraj/3(rideHard)
  DTFInput/1 -> Bus Selector1/1
  [groundSpd] -> ShapeRefTraj/2(gndSpd)
  Cos/1 -> Product/1
  Cast To Single/1 -> Add/2
  [wtp] -> Add/1
  Bus Selector/3 -> Mux/2  "<TRN_VelocityY>"
  [rideHardness] -> Bus Assignment2/2
  Mux/1 -> vectorNorm/1(u)
  Degrees to Radians/1 -> Cos/1
  Gain/1 -> Add1/2
  Add1/1 -> Cast To Single/1
  Bus Selector2/1 -> [wtp]  "<wtp>"
  TRNOutput/1 -> Bus Selector/1
  Add/1 -> ShapeRefTraj/1(refTraj)
  [TRNVerticalUncertainty] -> Gain/1
  vectorNorm/1(y) -> Product/2
  Bus Selector/2 -> Mux/1  "<TRN_VelocityX>"
  Bus Selector/4 -> Mux/3  "<TRN_VelocityZ>"
  pump/1 -> Bus Assignment1/1
  [msd] -> Bus Assignment2/3
  output/1 -> Bus Selector3/1, Bus Assignment2/1
  [msd] -> Add1/1
  Bus Selector/1 -> Degrees to Radians/1  "<TRN_Ver_FlightPath_Angle>"
  Bus Assignment2/1 -> output_/1
  Bus Selector1/1 -> [rideHardness]  "<rideQuality>"
  WTPGOutput/1 -> Bus Selector2/1
  Bus Assignment1/1 -> pump_/1
  Bus Selector3/1 -> [msd]  "<msdUsedWrap>"

== matlab function DTF/ImplementDTF/GenerateReferenceTrajectory/ShapeRefTraj ==
  data: shapedTraj output; refTraj input; gndSpd input; rideHard input
function shapedTraj = ShapeRefTraj(refTraj, gndSpd, rideHard)
%ShapeRefTraj
TRAJ_ALONG_STEPS          = 41;

% Initialize
shapedTraj      = zeros(TRAJ_ALONG_STEPS, 1, 'single');
slope           = zeros(TRAJ_ALONG_STEPS, 1);
hDiff           = 0.0;
upperG          = 0.0;
lowerG          = 0.0;
hUpThres        = 0.0;
hDownThres      = 0.0;
dt              = 0.5;
sweepingCount   = 0;

% Get Acceleration Limit
if (rideHard == 3)
    upperG = 2.0;
    lowerG = -0.9;    
elseif (rideHard == 2)
    upperG = 2.0;
    lowerG = -0.75;
elseif (rideHard == 1)
    upperG = 2.0;
    lowerG = -0.5;
else
    upperG = 2.0;
%     lowerG = -4.0;
    lowerG = -0.9;
end

% Calculate Threshold of Height Difference
hUpThres = (2*gndSpd^2 - sqrt(4*gndSpd^4-4*(upperG*9.8)^2*gndSpd^2*dt^2))/(2*(upperG*9.8));
hDownThres = (2*gndSpd^2 - sqrt(4*gndSpd^4-4*(lowerG*9.8)^2*gndSpd^2*dt^2))/(2*(lowerG*9.8));
Vmin = - gndSpd * sind(10);
Vmax = gndSpd * sind(30);
% 지시비행경로
Vmin = - gndSpd * sind(5);
Vmax = gndSpd * sind(5);

% Construct Slope and Reshape the Path
shapedTraj = refTraj;

while (sweepingCount < TRAJ_ALONG_STEPS*2)
    for ii = 1:TRAJ_ALONG_STEPS-1
        
        % Slope Calcuation
        if ii == 1
            slope(ii) = 0;
        elseif (ii > 5) && (ii < 37)
            slope(ii) = getVerticalSpeed(shapedTraj, 5, ii);
        else
            slope(ii) = (shapedTraj(ii+1)-shapedTraj(ii-1)) / (dt*2);
        end
        slope(ii) = saturate(slope(ii), Vmin, Vmax);

        hDiff = shapedTraj(ii+1) - shapedTraj(ii);
        
        if hDiff > (hUpThres + slope(ii)*dt)
            shapedTraj(ii) = shapedTraj(ii+1) - (hUpThres + slope(ii)*dt);
            sweepingCount = sweepingCount + 1;
        elseif (hDiff < hDownThres + slope(ii)*dt)
            shapedTraj(ii+1) = shapedTraj(ii) + (hDownThres + slope(ii)*dt);
        end
        
        if shapedTraj(ii) < refTraj(ii)
            shapedTraj(ii) = refTraj(ii);
            sweepingCount = sweepingCount + 1;
        end
    end
    sweepingCount = sweepingCount + 1;
end

end

%% sub function
function outVal = saturate(inVal, minVal, maxVal)
%saturate

% Initialize output
outVal = 0.0;

if (inVal > maxVal)
    outVal = maxVal;
elseif (inVal < minVal)
    outVal = minVal;
else
    outVal = inVal;
end

end

function vel = getVerticalSpeed(path, num, idx)

sum = single(0.0);
for i = 1:num
    sum = sum + single( (path(idx + i) - path(idx - i))/i );
end
vel = sum / single(num);

end

function vel = getVerticalSpeedInv(path, num, idx)

sum = 0;
for i = 1:num
    sum = sum + (path(idx - i) - path(idx + i))/i;
end
vel = sum / num;

end

== matlab function DTF/HandleDTFInput/SelectMsd ==
  data: msdPrev input; msdUse output; msdIn input
function msdUse = SelectMsd(msdPrev, msdIn)

msdUse = 0.0;


if ( (msdIn >= 15.24) && (msdIn <= 1524) )

    msdUse = msdIn;

else

    if ( (msdPrev >= 15.24) && (msdPrev <= 1524) )

        msdUse = msdPrev;

    else

        msdUse = 304.8;

    end

end

== matlab function DTF/ImplementDTF/GenerateReferenceTrajectory/vectorNorm ==
  data: u input; y output
function y = vectorNorm(u)
%VECTORNORM

y = norm(u);

== matlab function DTF/HandleDTFInput/CheckLowTF ==
  data: msdUse input; lowTF output; TRNEstHeightAGL input
function lowTF = CheckLowTF(msdUse, TRNEstHeightAGL)

lowTF = false;

if (TRNEstHeightAGL < 0.75*msdUse)

    lowTF = true;
end

end

== matlab function DTF/ImplementDTF/FollowReferenceTrajectory/CheckRideQuality ==
  data: rideQuality input; lookAheadTime output; upperG output; lowerG output
function [lookAheadTime, upperG, lowerG] = CheckRideQuality(rideQuality)
%CheckRideQuality
% 3.5 sec was best...

switch rideQuality
    case uint16(1)
        % Soft
        lookAheadTime = 3.5;
        upperG = 2.0;
        lowerG = -0.50;

    case uint16(2)
        % Medium
        lookAheadTime = 3.5;
        upperG = 2.0;
        lowerG = -0.75;

    case uint16(3)
        % Hard
        lookAheadTime = 3.5;
        upperG = 2.0;
        lowerG = -0.9;

    otherwise
        % Default (Not Used)
        lookAheadTime = 2.5;
        upperG = 2.0;
        lowerG = -4.00;
end

== matlab function DTF/ImplementDTF/FollowReferenceTrajectory/LimitGCommand ==
  data: rawGCmd input; gCmd output; setWarnG output; upperG input; lowerG input
function [gCmd, setWarnG] = LimitGCommand(rawGCmd, upperG, lowerG)
%LIMITGCOMMAND
% Limit G Command Upper/Lower Bounds

% Initialize Outputs
gCmd    = 0.0;
setWarnG    = false;

% Saturate and Check G Warinng
if (rawGCmd > upperG)
    gCmd = upperG;
    setWarnG = true;
elseif (rawGCmd < lowerG)
    gCmd = lowerG;
    setWarnG = false;
else
    gCmd = rawGCmd;
    setWarnG = false;
end

== matlab function DTF/ImplementDTF/FollowReferenceTrajectory/ConvertBody2NED ==
  data: eulerDeg input; vecNED output; vecXYZ input; C_b_n output
function [vecNED, C_b_n] = ConvertBody2NED(eulerDeg, vecXYZ)
%ConvertBody2NED 동체 좌표계 벡터를 NED 좌표계 벡터로 변환
% Body2NED 변환 행렬 출력

% Initialize
vecNED = zeros(3,1);
C_n_b = zeros(3,3);
C_b_n = zeros(3,3);

% Trigonometirc functions
cRol = cosd(eulerDeg(1));
sRol = sind(eulerDeg(1));
cPit = cosd(eulerDeg(2));
sPit = sind(eulerDeg(2));
cYaw = cosd(eulerDeg(3));
sYaw = sind(eulerDeg(3));

% Transformation matrix
C_n_b   = [              cPit*cYaw,                cPit*sYaw,     -sPit;...
          sRol*sPit*cYaw-cRol*sYaw, sRol*sPit*sYaw+cRol*cYaw, sRol*cPit;...
          cRol*sPit*cYaw+sRol*sYaw, cRol*sPit*sYaw-sRol*cYaw, cRol*cPit];

C_b_n   = C_n_b';

% Transform
vecNED = C_b_n * vecXYZ;

end

== matlab function DTF/ImplementDTF/FollowReferenceTrajectory/GenerateTFCommand ==
  data: refPath input; velNED input; llh input; accXYZ input; pitch input; lookAheadTime input; gCommand output
function gCommand  = GenerateTFCommand(refPath, velNED, llh, accXYZ, pitch, lookAheadTime)
%GENERATETFCOMMAND 지형추적을 위한 수직가속도 명령 생성
% Initialize
diffH = 0.0;
dist = 0.0;
lookAhead = 0.0;
gndSpd = 0.0;
radius = 0.0;

%% [1] Handle Inputs and Define Constants
velN    = velNED(1);
velE    = velNED(2);
velU    = -velNED(3);

% Ground Speed
gndSpd  = sqrt( velE^2 + velN^2 );
gndSpd  = saturate(gndSpd, 75.1089, 360.111);

lat     = llh(1);
lon     = llh(2);
alt     = llh(3);

% Initialize Outputs
gCommand    = 0.0;
gain        = 1.0;
radius      = 0.0;
idx         = 0;

% Scan Interval
dt          = 0.5;

%% [2] Check Ride Hardness

%% [3] Generate G Command

% Sweeping interval (distance range of neighbor)
sweepInterval   = 1;

% Sweeping Interval
sweepNum        = 1 + 2*sweepInterval;

% Candidate for any pull-up required in neighboring index
temp = zeros(3,sweepNum);

% Check any pull-up required in the sweeping interval
radiusSignFlag  = false;

% Pseudo/Approximated Acc Up
pseudoAccU      = accXYZ(1) * sind(pitch) - accXYZ(3) * cosd(pitch);

for ii = 1:sweepNum
    % lookAhead: The height of lookAhead point. "double" used since refPath is single
    time        = lookAheadTime + (ii - 1 - sweepInterval) * dt;
    lookAhead   = getLookAheadHeight(refPath, time);

    % diffH: Effective vertical distance. ( diffH > 0 : Aircraft is lower )
    diffH       = double ( lookAhead ) - alt ...
                - velU * (time ) ...
                - 0.5 * pseudoAccU * ( dt )^2;

    % Horizontal distance
    dist        = gndSpd * time;

    % Detour for divide by zero
    diffH = sign(diffH) * saturate(abs(diffH), 0.1, abs(dist));

    % Radius of curvautre
    radius      = ( diffH / 2 ) + ( dist^2 ) / ( 2*diffH );
    
    temp(1,ii)  = radius;
    temp(2,ii)  = diffH;
    
    % If any pull-up required ?
    radiusSignFlag = (radius >= 0);

end

% Choose worst case
[radius, idx] = min(temp(1,:));

if (radiusSignFlag)
    for jj = 1:sweepNum
        if temp(1,jj) >= 0
            temp(3,jj) = temp(1,jj);
        else
            temp(3,jj) = max(temp(1,:));
        end
    end
    radius = min(temp(3,:));
end

gain    = 1.0;
% Udershoot rejection gain is disabled
% if temp(2, idx) < 0
%     gain = 1.0;
% end

gCommand = (gain * gndSpd^2 / radius) / 9.807;

end
%% --- Internal Functions
function outVal = saturate(inVal, minVal, maxVal)
%saturate

% Initialize output
outVal = 0.0;

outVal = min(maxVal, max(minVal, inVal));

end

function height = getLookAheadHeight(refTraj, time)
%getLookAheadHeight

% Initialize output
height = 0.0;

dt = 0.5;

idx1 = floor(1 + time/dt);
idx2 = ceil(1 + time/dt);

height = (1 - mod(time, dt)/dt) * refTraj(idx1) ...
    + mod(time, dt)/dt * refTraj(idx2);

end
